simulink model "slo_delay_bal"  (R2015b)
settings: Solver=FixedStepDiscrete  SolverMode=SingleTasking  StartTime=0.0  StopTime=10  RelTol=1e-3
libraries: simulink x2
CloseFcn:
  | rtwprivate ssgencode ModelCloseRequest Hysteresis_test1
settings Model: DataTypeOverride=Off  Creator=at-mt  LastModifiedBy=amatsumo
settings DataIOCC: SaveFormat=Array  SaveOutput=off  SignalLogging=off  SaveTime=off
settings OptimizationCC: BlockReduction=off  ConditionallyExecuteInputs=off  DefaultParameterBehavior=Inlined  ExpressionDepthLimit=2147483647
settings DebuggingCC: AlgebraicLoopMsg=error  UnderspecifiedInitializationDetection=Classic  MergeDetectMultiDrivingBlocksExec=none  SolverPrmCheckMsg=warning  SingleTaskRateTransMsg=error  FcnCallInpInsideContextMsg=UseLocalSettings  StateNameClashWarn=warning
settings HardwareCC: ProdBitPerPointer=32  ProdLargestAtomicFloat=None  ProdIntDivRoundTo=Undefined  ProdEndianess=Unspecified  ProdWordSize=32  ProdHWDeviceType=ASIC/FPGA->ASIC/FPGA  ProdEqTarget=off
settings GRTTargetCC: GeneratePreprocessorConditionals=Disable all  CombineOutputUpdateFcns=off  GRTInterface=on
settings ConfigComp: CovModelRefEnable=Off  CovSFcnEnable=off

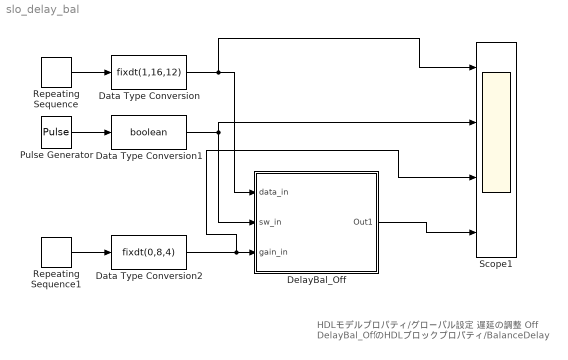
== system slo_delay_bal ==
  note: HDLモデルプロパティ/グローバル設定
      | 遅延の調整 Off
      | DelayBal_OffのHDLブロックプロパティ/BalanceDelay
  Data Type Conversion : DataTypeConversion  OutMin=0  OutMax=2*pi  OutDataTypeStr=fixdt(1,16,12)  SampleTime=1/1000
  Data Type Conversion1 : DataTypeConversion  OutDataTypeStr=boolean  SampleTime=1/1000
  Data Type Conversion2 : DataTypeConversion  OutMin=0  OutMax=10  OutDataTypeStr=fixdt(0,8,4)  SampleTime=1/1000
  DelayBal_Off : Subsystem
  Pulse Generator : DiscretePulseGenerator  Period=1000*10  PulseWidth=1000*5  SampleTime=1/1000
  Repeating Sequence : simulink/Sources/Repeating Sequence  rep_seq_t=[0 5]  rep_seq_y=[0 2*pi]*0.999
  Repeating Sequence1 : simulink/Sources/Repeating Sequence  rep_seq_t=[0 4.999 5 7.999 8 10]  rep_seq_y=[2 2 5 5 3 3]
  Scope1 : Scope  NumInputPorts=4
  wires:
  Repeating Sequence/1 -> Data Type Conversion/1
  Pulse Generator/1 -> Data Type Conversion1/1
  Data Type Conversion1/1 -> DelayBal_Off/2(sw_in), Scope1/2
  Repeating Sequence1/1 -> Data Type Conversion2/1
  Data Type Conversion2/1 -> Scope1/3, DelayBal_Off/3(gain_in)
  Data Type Conversion/1 -> Scope1/1, DelayBal_Off/1(data_in)
  DelayBal_Off/1(Out1) -> Scope1/4

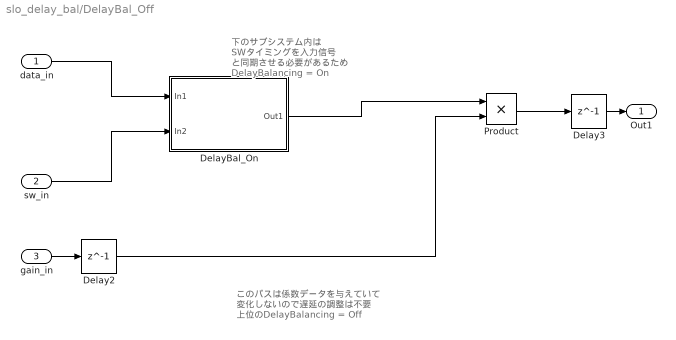
== system slo_delay_bal/DelayBal_Off ==
  note: このパスは係数データを与えていて
      | 変化しないので遅延の調整は不要
      | 上位のDelayBalancing = Off
  note: 下のサブシステム内は
      | SWタイミングを入力信号
      | と同期させる必要があるため
      | DelayBalancing = On
  data_in : Inport
  sw_in : Inport  Port=2
  gain_in : Inport  Port=3
  Delay2 : Delay  DelayLength=1
  Delay3 : Delay  DelayLength=1
  DelayBal_On : Subsystem
  Product : Product  RndMeth=Zero
  Out1 : Outport
  wires:
  Delay3/1 -> Out1/1
  gain_in/1 -> Delay2/1
  Product/1 -> Delay3/1
  Delay2/1 -> Product/2
  data_in/1 -> DelayBal_On/1(In1)
  sw_in/1 -> DelayBal_On/2(In2)
  DelayBal_On/1(Out1) -> Product/1

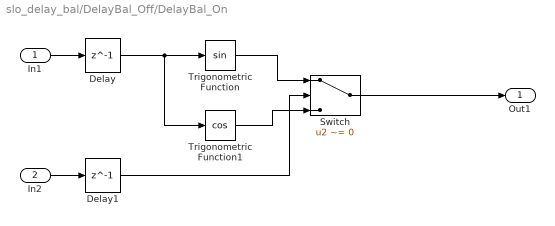
== system slo_delay_bal/DelayBal_Off/DelayBal_On ==
  In1 : Inport
  In2 : Inport  Port=2
  Delay : Delay  DelayLength=1
  Delay1 : Delay  DelayLength=1
  Switch : Switch  Criteria=u2 ~= 0
  Trigonometric Function : Trigonometry  ApproximationMethod=CORDIC
  Trigonometric Function1 : Trigonometry  Operator=cos  ApproximationMethod=CORDIC
  Out1 : Outport
  wires:
  Trigonometric Function/1 -> Switch/1
  Trigonometric Function1/1 -> Switch/3
  Delay1/1 -> Switch/2
  Switch/1 -> Out1/1
  In2/1 -> Delay1/1
  Delay/1 -> Trigonometric Function1/1, Trigonometric Function/1
  In1/1 -> Delay/1
